simulink model "scara"  (R2015a)
settings: Solver=ode1  StartTime=0.0  StopTime=Inf  FixedStep=0.001  RelTol=1e-3
PostLoadFcn:
  | , if any(exist('dsrtsu_mdlpostloadfcn', 'file') == [2, 3, 6]), try dsrtsu_mdlpostloadfcn('Execute', bdroot); catch fprintf('Error in PostLoadFcn (dsrtsu_mdlpostloadfcn) for model "%s":\n %s\n', bdroot, lasterr); end, end,
libraries: rtilib1104 x9, simulink x6, simulink_extras x4
settings Model: DSRTSU_INTERNAL_RTI_VER=460  DSRTSU_INTERNAL_RTI_TYPE=rti1104  DSRTSU_INTERNAL_RTIFPGA=50  Creator=k21c900a  LastModifiedBy=k21c900a
settings OptimizationCC: BlockReduction=off  OptimizeBlockIOStorage=off  BufferReuse=off  GlobalBufferReuse=off  ExpressionFolding=off  LocalBlockOutputs=off
settings HardwareCC: ProdIntDivRoundTo=Zero  ProdEndianess=BigEndian  ProdHWDeviceType=Generic->Custom  TargetIntDivRoundTo=Zero  TargetEndianess=BigEndian  TargetHWDeviceType=Generic->Custom
settings RTWCC: SystemTargetFile=rti1104.tlc  MakeCommand=make_rti  TemplateMakefile=rti1104.tmf  Description=dSPACE DS1104 Hardware Platform
settings STFCustomTargetCC: GenerateSampleERTMain=off  ParMdlRefBuildCompliant=on  GeneratePreprocessorConditionals=Disable all  ERTCustomFileBanners=off  SupportNonInlinedSFcns=on  SupportVariableSizeSignals=off  MATLABClassNameForMDSCustomization=Simulink.SoftwareTarget.GRTCustomization  GRTInterface=on  SystemTargetFile=rti1104.tlc
settings GRTTargetCC: CompOptLevelCompliant=off  ConcurrentExecutionCompliant=off  CombineOutputUpdateFcns=off  MatFileLogging=off  CPPClassGenCompliant=off  GRTInterface=on  ExtModeMexFile=noextcomm

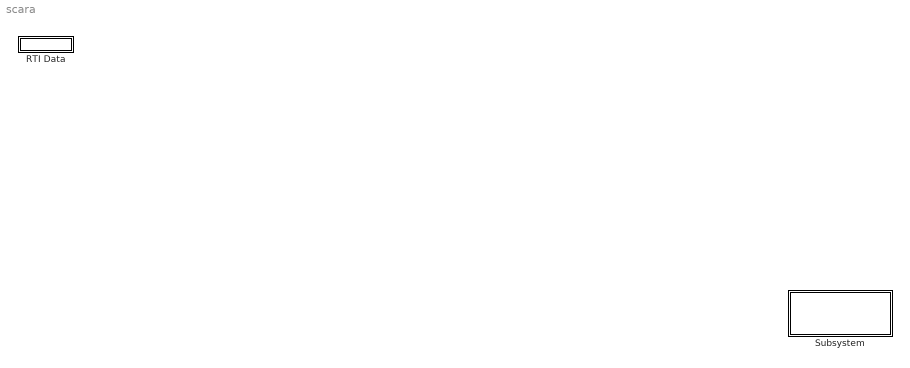
== system scara ==
  RTI Data : Subsystem  Tag=struct('RTIDataServer',struct('RTIDataServerVs','2','RTIModelDescription','struct(''main'',''scara'',''sub'','''',''isMp'',0)'))  LoadFcn="if exist('rtidc'), try,  rtidc('DataHostBlockClbLoad', gcbh); catch, disp(['Warning: ''LoadFcn'' for RTI Data block failed: ' lasterr]); end, end,"  mask(RTI_DATA_HOST){}
      mask help:
      | RTI Data Block.
      | This block is used by RTI to store internal model-dependent data.
      | Please keep this block on the root level of the model. Deleting this block will result in data loss.
      |
      | NEVER DELETE OR COPY THIS BLOCK!
      settings: CopyFcn="if exist('rtidc'), try,  rtidc('DataHostBlockClbCopy', gcbh); catch, disp(['Warning: ''CopyFcn'' for RTI Data block failed: ' lasterr]); end, end,"  DeleteFcn="if exist('rtidc'), try,  rtidc('DataHostBlockClbDelete', gcbh); catch, disp(['Warning: ''DeleteFcn'' for RTI Data block failed: ' lasterr]); end, end,"  ModelCloseFcn="if exist('rtidc'), try,  rtidc('DataHostBlockClbModelClose', gcbh); catch, disp(['Warning: ''ModelCloseFcn'' for RTI Data block failed: ' lasterr]); end, end,"  PreSaveFcn="if exist('rtidc'), try,  rtidc('DataHostBlockClbPreSave', gcbh); catch, disp(['Warning: ''PreSaveFcn'' for RTI Data block failed: ' lasterr]); end, end,"  PostSaveFcn="if exist('rtidc'), try,  rtidc('DataHostBlockClbPostSave', gcbh); catch, disp(['Warning: ''PostSaveFcn'' for RTI Data block failed: ' lasterr]); end, end,"  NameChangeFcn="if exist('rtidc'), try,  rtidc('DataHostBlockClbNameChange', gcbh); catch, disp(['Warning: ''NameChangeFcn'' for RTI Data block failed: ' lasterr]); end, end,"
      mask Help:
      | RTI Data Block.
      | This block is used by RTI to store internal model-dependent data.
      | Please keep this block on the root level of the model. Deleting this block will result in data loss.
      | 
      | NEVER DELETE OR COPY THIS BLOCK!
      mask Display:
      | text(0.5, 0.5, 'RTI Data', 'HorizontalAlignment', 'center');
      | plot([1 0]);
  Subsystem : Subsystem

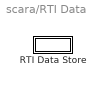
== system scara/RTI Data ==
  RTI Data Store : Subsystem  Tag="struct('private',struct('version',struct('dsVer',uint32(2),'dsVerCreation',uint32(2),'RTI',struct('ver','7.4','type','RTI1104')),'access',struct('type','Model','isPerm',1,'created',['18-Nov-2021 09:18:31'],'modified',['25-Nov-2021 10:31:28'],'location','')),'public',struct('main',struct('data',[]),'sub',struct('name',{{'scara'}},'data',{{struct('TH',struct('thTaskInfo',struct('taskType',{'TIMER','HWINT','TMRINT','SWINT','GLINT'},'tasksNumOf',{1,0,0,0,0},'srcIds',{{'TIMERA'},{},{},{},{}},'taskNames',{{['Timer Task 1']},{},{},{},{}})),'th_tc',struct('dataType','TASK','taskGroupId','','taskGroupList',{{}},'taskSchedulingPolicy','FCFS','taskType','TIMER','blkh',-1,'srcId','TIMERA','srcSgnName',['Timer A interrupt'],'srcCpuName','','taskName',['Timer Task 1  [0.001] s'],'taskNameDisplayExt','','smplTime',0.001,'smplTimeOffs',0,'hasFixedPriority',0,'priority',1,'hasFixedOvc',0,'ovcType',1,'ovcMax',1),'tc_th',struct('dataType','TASK','taskGroupId','','taskGroupList',{{}},'taskSchedulingPolicy','FCFS','taskType','TIMER','blkh',-1,'srcId','TIMERA','srcSgnName',['Timer A interrupt'],'srcCpuName','','taskName',['Timer Task 1  [0.001] s'],'taskNameDisplayExt','','smplTime',0.001,'smplTimeOffs',0,'hasFixedPriority',0,'priority',1,'hasFixedOvc',0,'ovcType',1,'ovcMax',1))}})))"  mask(RTI_DATA_STORE){}
      mask help:
      | RTI Data Store Block. This block is used by RTI to store internal model dependent data. Deleting this block will result in data loss.
      |
      | NEVER DELETE, COPY, OR MODIFY THIS BLOCK!
      mask Help:
      | RTI Data Store Block. This block is used by RTI to store internal model dependent data. Deleting this block will result in data loss.
      | 
      | NEVER DELETE, COPY, OR MODIFY THIS BLOCK!
      mask Display: text(0.5, 0.5, ' ', 'HorizontalAlignment', 'center');

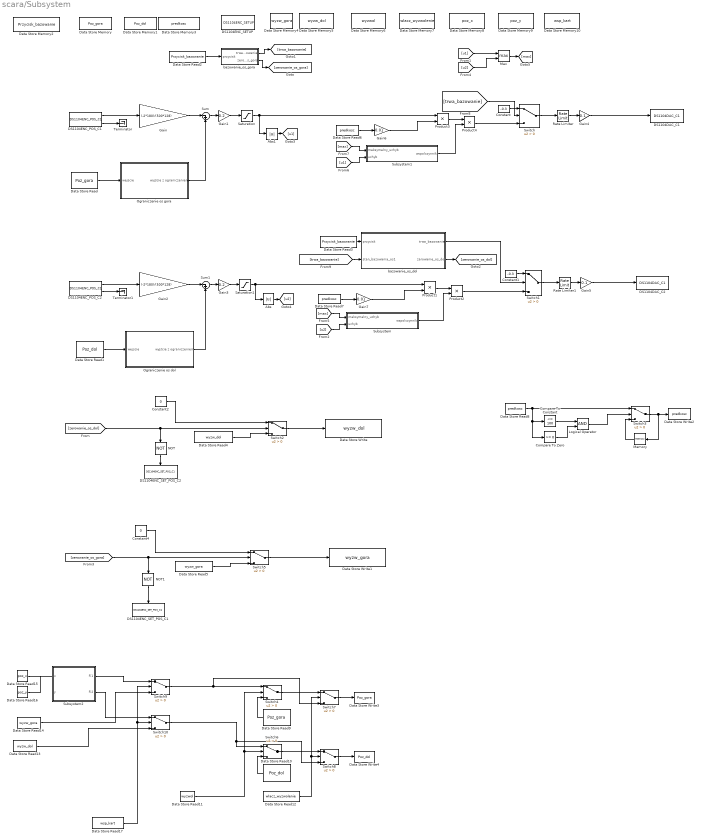
== system scara/Subsystem ==
  Abs : Abs
  Abs1 : Abs
  Compare To Constant : simulink/Logic and Bit Operations/Compare To Constant  relop=<=  const=100  OutDataTypeStr=boolean
  Compare To Zero : simulink/Logic and Bit Operations/Compare To Zero  relop=>=  OutDataTypeStr=boolean
  Constant : Constant  Value=-0.3
  Constant1 : Constant  Value=-0.3
  Constant2 : Constant  Value=0
  Constant4 : Constant  Value=0
  DS1104DAC_C1 : rtilib1104/DS1104 MASTER PPC/DS1104DAC_C1  ChannelNo=1  InitValue=0  TermMode=0  TermValue=0  Reserved1=[]  Reserved2=[]  Reserved3=[]  Reserved4=[]  DialogFcn=gui1104dac  UnitName={ 'DS1104DAC_C'}  UnitValues={ 1 }  DSProperties=struct('RTI',struct('Version',uint32(1),'BlockType',struct('isSLSource',uint8(0),'isSLSink',uint8(1),'isHWSource',uint8(0),'isHWSink',uint8(1),'isSetup',uint8(0),'isInline',uint8(1),'isNonInline',uint8(0),'isInterrupt',uint8(0),'isChannelwise',uint8(1)),'IOBoardType','DS1104MASTER','UnitType','DAC','Identifier','DAC','DialogType','ML','BlockSet','NONE','SlaveProcessor','NONE'))
  DS1104DAC_C2 : rtilib1104/DS1104 MASTER PPC/DS1104DAC_C1  ChannelNo=2  InitValue=0  TermMode=0  TermValue=0  Reserved1=[]  Reserved2=[]  Reserved3=[]  Reserved4=[]  DialogFcn=gui1104dac  UnitName={ 'DS1104DAC_C'}  UnitValues={2}  DSProperties=struct('RTI',struct('Version',uint32(1),'BlockType',struct('isSLSource',uint8(0),'isSLSink',uint8(1),'isHWSource',uint8(0),'isHWSink',uint8(1),'isSetup',uint8(0),'isInline',uint8(1),'isNonInline',uint8(0),'isInterrupt',uint8(0),'isChannelwise',uint8(1)),'IOBoardType','DS1104MASTER','UnitType','DAC','Identifier','DAC','DialogType','ML','BlockSet','NONE','SlaveProcessor','NONE'))
  DS1104ENC_POS_C1 : rtilib1104/DS1104 MASTER PPC/DS1104ENC_POS_C1  ChannelNo=1  PosValue=0  Reserved1=[]  Reserved2=[]  Reserved3=[]  Reserved4=[]  DialogFcn=gui1104enc_pos  UnitName={'DS1104ENC_POS_C'}  UnitValues={ 1 }  DSProperties=struct('RTI',struct('Version',uint32(1),'BlockType',struct('isSLSource',uint8(1),'isSLSink',uint8(0),'isHWSource',uint8(1),'isHWSink',uint8(0),'isSetup',uint8(0),'isInline',uint8(1),'isNonInline',uint8(0),'isInterrupt',uint8(0),'isChannelwise',uint8(1)),'IOBoardType','DS1104MASTER','UnitType','ENC','Identifier','ENCPOSCH','DialogType','ML','BlockSet','NONE','SlaveProcessor','NONE'))
  DS1104ENC_POS_C2 : rtilib1104/DS1104 MASTER PPC/DS1104ENC_POS_C1  ChannelNo=2  PosValue=0  Reserved1=[]  Reserved2=[]  Reserved3=[]  Reserved4=[]  DialogFcn=gui1104enc_pos  UnitName={'DS1104ENC_POS_C'}  UnitValues={2}  DSProperties=struct('RTI',struct('Version',uint32(1),'BlockType',struct('isSLSource',uint8(1),'isSLSink',uint8(0),'isHWSource',uint8(1),'isHWSink',uint8(0),'isSetup',uint8(0),'isInline',uint8(1),'isNonInline',uint8(0),'isInterrupt',uint8(0),'isChannelwise',uint8(1)),'IOBoardType','DS1104MASTER','UnitType','ENC','Identifier','ENCPOSCH','DialogType','ML','BlockSet','NONE','SlaveProcessor','NONE'))
  DS1104ENC_SETUP : rtilib1104/DS1104 MASTER PPC/DS1104ENC_SETUP  Reserved1=[]  Reserved2=[]  Reserved3=[]  Reserved4=[]  DialogFcn=gui1104enc_setup  UnitName={'DS1104ENC_SETUP'}  UnitValues={ [] }  DSProperties=struct('RTI',struct('Version',uint32(1),'BlockType',struct('isSLSource',uint8(0),'isSLSink',uint8(0),'isHWSource',uint8(0),'isHWSink',uint8(0),'isSetup',uint8(0),'isInline',uint8(1),'isNonInline',uint8(0),'isInterrupt',uint8(0),'isChannelwise',uint8(0)),'IOBoardType','DS1104MASTER','UnitType','ENC','Identifier','ENCSETUP','DialogType','ML','BlockSet','NONE','SlaveProcessor','NONE'))
      settings: SignalType=[0 0]
  DS1104ENC_SET_POS_C1 : rtilib1104/DS1104 MASTER PPC/DS1104ENC_SET_POS_C1  ChannelNo=1  PosValue=0  Reserved1=[]  Reserved2=[]  Reserved3=[]  Reserved4=[]  DialogFcn=gui1104enc_set_pos  UnitName={'DS1104ENC_SET_POS_C'}  UnitValues={ 1 }  DSProperties=struct('RTI',struct('Version',uint32(1),'BlockType',struct('isSLSource',uint8(0),'isSLSink',uint8(1),'isHWSource',uint8(0),'isHWSink',uint8(1),'isSetup',uint8(0),'isInline',uint8(1),'isNonInline',uint8(0),'isInterrupt',uint8(0),'isChannelwise',uint8(1)),'IOBoardType','DS1104MASTER','UnitType','ENC','Identifier','ENCRESET','DialogType','ML','BlockSet','NONE','SlaveProcessor','NONE'))
  DS1104ENC_SET_POS_C2 : rtilib1104/DS1104 MASTER PPC/DS1104ENC_SET_POS_C1  ChannelNo=2  PosValue=0  Reserved1=[]  Reserved2=[]  Reserved3=[]  Reserved4=[]  DialogFcn=gui1104enc_set_pos  UnitName={'DS1104ENC_SET_POS_C'}  UnitValues={ 2 }  DSProperties=struct('RTI',struct('Version',uint32(1),'BlockType',struct('isSLSource',uint8(0),'isSLSink',uint8(1),'isHWSource',uint8(0),'isHWSink',uint8(1),'isSetup',uint8(0),'isInline',uint8(1),'isNonInline',uint8(0),'isInterrupt',uint8(0),'isChannelwise',uint8(1)),'IOBoardType','DS1104MASTER','UnitType','ENC','Identifier','ENCRESET','DialogType','ML','BlockSet','NONE','SlaveProcessor','NONE'))
  Data Store Memory : DataStoreMemory  DataStoreName=Poz_gora  ReadBeforeWriteMsg=warning  WriteAfterWriteMsg=warning  WriteAfterReadMsg=warning
  Data Store Memory1 : DataStoreMemory  DataStoreName=Poz_dol  ReadBeforeWriteMsg=warning  WriteAfterWriteMsg=warning  WriteAfterReadMsg=warning
  Data Store Memory10 : DataStoreMemory  DataStoreName=wsp_kart  ReadBeforeWriteMsg=warning  WriteAfterWriteMsg=warning  WriteAfterReadMsg=warning
  Data Store Memory2 : DataStoreMemory  DataStoreName=Przycisk_bazowanie  ReadBeforeWriteMsg=warning  WriteAfterWriteMsg=warning  WriteAfterReadMsg=warning
  Data Store Memory3 : DataStoreMemory  DataStoreName=predkosc  ReadBeforeWriteMsg=warning  WriteAfterWriteMsg=warning  WriteAfterReadMsg=warning
  Data Store Memory4 : DataStoreMemory  DataStoreName=wyzw_gora  ReadBeforeWriteMsg=warning  WriteAfterWriteMsg=warning  WriteAfterReadMsg=warning
  Data Store Memory5 : DataStoreMemory  DataStoreName=wyzw_dol  ReadBeforeWriteMsg=warning  WriteAfterWriteMsg=warning  WriteAfterReadMsg=warning
  Data Store Memory6 : DataStoreMemory  DataStoreName=wyzwol  ReadBeforeWriteMsg=warning  WriteAfterWriteMsg=warning  WriteAfterReadMsg=warning
  Data Store Memory7 : DataStoreMemory  DataStoreName=wlacz_wyzwolenie  ReadBeforeWriteMsg=warning  WriteAfterWriteMsg=warning  WriteAfterReadMsg=warning
  Data Store Memory8 : DataStoreMemory  DataStoreName=poz_x  ReadBeforeWriteMsg=warning  WriteAfterWriteMsg=warning  WriteAfterReadMsg=warning
  Data Store Memory9 : DataStoreMemory  DataStoreName=poz_y  ReadBeforeWriteMsg=warning  WriteAfterWriteMsg=warning  WriteAfterReadMsg=warning
  Data Store Read : DataStoreRead  DataStoreName=Poz_gora
  Data Store Read1 : DataStoreRead  DataStoreName=Poz_dol
  Data Store Read10 : DataStoreRead  DataStoreName=Poz_dol
  Data Store Read11 : DataStoreRead  DataStoreName=wyzwol
  Data Store Read12 : DataStoreRead  DataStoreName=wlacz_wyzwolenie
  Data Store Read13 : DataStoreRead  DataStoreName=wyzw_dol
  Data Store Read14 : DataStoreRead  DataStoreName=wyzw_gora
  Data Store Read15 : DataStoreRead  DataStoreName=poz_x
  Data Store Read16 : DataStoreRead  DataStoreName=poz_y
  Data Store Read17 : DataStoreRead  DataStoreName=wsp_kart
  Data Store Read2 : DataStoreRead  DataStoreName=Przycisk_bazowanie
  Data Store Read3 : DataStoreRead  DataStoreName=Przycisk_bazowanie
  Data Store Read4 : DataStoreRead  DataStoreName=wyzw_dol
  Data Store Read5 : DataStoreRead  DataStoreName=wyzw_gora
  Data Store Read6 : DataStoreRead  DataStoreName=predkosc
  Data Store Read7 : DataStoreRead  DataStoreName=predkosc
  Data Store Read8 : DataStoreRead  DataStoreName=predkosc
  Data Store Read9 : DataStoreRead  DataStoreName=Poz_gora
  Data Store Write : DataStoreWrite  DataStoreName=wyzw_dol
  Data Store Write1 : DataStoreWrite  DataStoreName=wyzw_gora
  Data Store Write2 : DataStoreWrite  DataStoreName=predkosc
  Data Store Write3 : DataStoreWrite  DataStoreName=Poz_gora
  Data Store Write4 : DataStoreWrite  DataStoreName=Poz_dol
  Gain : Gain  Gain=(-2*180)/(500*128)
  Gain1 : Gain  Gain=0.2
  Gain2 : Gain  Gain=(-2*180)/(500*128)
  Gain3 : Gain  Gain=0.2
  Gain4 : Gain  Gain=0.1
  Gain5 : Gain  Gain=0.1
  Gain6 : Gain  Gain=0.01
  Gain7 : Gain  Gain=0.01
  Logical Operator : Logic  AllPortsSameDT=off  OutDataTypeStr=boolean
  Max : MinMax  Function=max  Inputs=2
  Memory : Memory
  NOT : Logic  Operator=NOT  IconShape=distinctive  AllPortsSameDT=off  OutDataTypeStr=boolean
  NOT1 : Logic  Operator=NOT  IconShape=distinctive  AllPortsSameDT=off  OutDataTypeStr=boolean
  Ograniczenie os dol : Subsystem
  Ograniczenie os gora : Subsystem
  Product{1..4} (4 alike) : Product
  Rate Limiter : RateLimiter  RisingSlewLimit=50  FallingSlewLimit=-50  SampleTimeMode=inherited
  Rate Limiter1 : RateLimiter  RisingSlewLimit=50  FallingSlewLimit=-50  SampleTimeMode=inherited
  Saturation : Saturate  UpperLimit=3  LowerLimit=-3
  Saturation1 : Saturate  UpperLimit=3  LowerLimit=-3
  Subsystem : Subsystem
  Subsystem1 : Subsystem
  Subsystem2 : Subsystem
  Sum : Sum  Inputs=|-+
  Sum1 : Sum  Inputs=|-+
  Switch{,1..10} (11 alike) : Switch  Criteria=u2 > Threshold
  Terminator : Terminator
  Terminator1 : Terminator
  bazowanie_os_dol : Subsystem
  bazowanie_os_gora : Subsystem
  wires:
  Data Store Read2/1 -> bazowanie_os_gora/1(przycisk)
  Data Store Read4/1 -> Switch2/3
  Switch2/1 -> Data Store Write/1
  [zerowanie_os_dol] -> Switch2/2, NOT/1
  Constant2/1 -> Switch2/1
  NOT/1 -> DS1104ENC_SET_POS_C2/Trigger
  bazowanie_os_gora/2(zerowanie_os_gora) -> [zerowanie_os_gora]
  bazowanie_os_gora/1(trwa_bazowanie) -> [trwa_bazowanie]
  Switch5/1 -> Data Store Write1/1
  Constant4/1 -> Switch5/1
  Data Store Read5/1 -> Switch5/3
  [zerowanie_os_gora] -> NOT1/1, Switch5/2
  NOT1/1 -> DS1104ENC_SET_POS_C1/Trigger
  DS1104ENC_POS_C1/2 -> Terminator/1
  DS1104ENC_POS_C1/1 -> Gain/1
  Gain/1 -> Sum/1
  Sum/1 -> Gain1/1
  Rate Limiter/1 -> Gain4/1
  DS1104ENC_POS_C2/2 -> Terminator1/1
  DS1104ENC_POS_C2/1 -> Gain2/1
  Gain2/1 -> Sum1/1
  Sum1/1 -> Gain3/1
  Gain3/1 -> Saturation1/1
  Rate Limiter1/1 -> Gain5/1
  Data Store Read/1 -> Ograniczenie os gora/1(wejscie)
  Ograniczenie os gora/1(wyjście z ograniczeniem) -> Sum/2
  Data Store Read1/1 -> Ograniczenie os dol/1(wejscie)
  Ograniczenie os dol/1(wyjście z ograniczeniem) -> Sum1/2
  Gain4/1 -> DS1104DAC_C1/1
  Gain5/1 -> DS1104DAC_C2/1
  Gain1/1 -> Saturation/1
  Constant/1 -> Switch/1
  Switch/1 -> Rate Limiter/1
  Constant1/1 -> Switch1/1
  bazowanie_os_dol/1(trwa_bazowanie) -> Switch1/2
  Switch1/1 -> Rate Limiter1/1
  Data Store Read3/1 -> bazowanie_os_dol/1(przycisk)
  bazowanie_os_dol/2(zarowanie_os_dol) -> [zerowanie_os_dol]
  Abs1/1 -> [u1]
  Abs/1 -> [u2]
  Product1/1 -> Product2/1
  Saturation1/1 -> Product1/1, Abs/1
  Subsystem/1(wspolczynnik) -> Product2/2
  [u2] -> Subsystem/2(uchyb)
  Product2/1 -> Switch1/3
  Data Store Read7/1 -> Gain7/1
  Gain7/1 -> Product1/2
  [max] -> Subsystem/1(maksymalny_uchyb)
  Product3/1 -> Product4/1
  Saturation/1 -> Product3/1, Abs1/1
  Subsystem1/1(wspolczynnik) -> Product4/2
  [u1] -> Subsystem1/2(uchyb)
  Product4/1 -> Switch/3
  Data Store Read6/1 -> Gain6/1
  Gain6/1 -> Product3/2
  [max] -> Subsystem1/1(maksymalny_uchyb)
  [trwa_bazowanie] -> Switch/2
  [trwa_bazowanie] -> bazowanie_os_dol/2(stan_bazowania_os1)
  [u1] -> Max/1
  [u2] -> Max/2
  Max/1 -> [max]
  Switch3/1 -> Memory/1, Data Store Write2/1
  Memory/1 -> Switch3/3
  Data Store Read8/1 -> Compare To Constant/1, Compare To Zero/1, Switch3/1
  Compare To Constant/1 -> Logical Operator/1
  Compare To Zero/1 -> Logical Operator/2
  Logical Operator/1 -> Switch3/2
  Data Store Read11/1 -> Switch6/2, Switch4/2
  Switch4/1 -> Switch7/1
  Switch6/1 -> Switch8/1
  Data Store Read12/1 -> Switch8/2, Switch7/2
  Data Store Read9/1 -> Switch4/3
  Data Store Read10/1 -> Switch6/3
  Switch7/1 -> Data Store Write3/1
  Switch8/1 -> Data Store Write4/1
  Switch9/1 -> Switch7/3, Switch4/1
  Switch10/1 -> Switch6/1, Switch8/3
  Data Store Read15/1 -> ?
  Data Store Read16/1 -> ?
  Data Store Read17/1 -> Switch9/2, Switch10/2
  Data Store Read14/1 -> Switch9/3
  Data Store Read13/1 -> Switch10/3
  Subsystem2/1(Fi1) -> Switch9/1
  Subsystem2/2(Fi2) -> Switch10/1

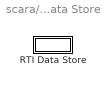
== system scara/RTI Data/RTI Data Store ==
  RTI Data Store : Subsystem  mask(RTI_DATA_STORE){}
      mask help:
      | RTI Data Store Block. This block is used by RTI to store internal model dependent data. Deleting this block will result in data loss.
      |
      | NEVER DELETE, COPY, OR MODIFY THIS BLOCK!
      mask Help:
      | RTI Data Store Block. This block is used by RTI to store internal model dependent data. Deleting this block will result in data loss.
      | 
      | NEVER DELETE, COPY, OR MODIFY THIS BLOCK!
      mask Display: text(0.5, 0.5, ' ', 'HorizontalAlignment', 'center');

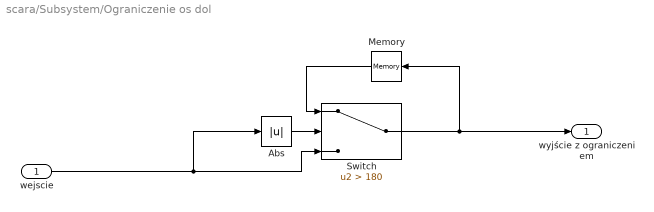
== system scara/Subsystem/Ograniczenie os dol ==
  wejscie : Inport
  Abs : Abs
  Memory : Memory
  Switch : Switch  Criteria=u2 > Threshold  Threshold=180
  wyjście z ograniczeniem : Outport
  wires:
  Memory/1 -> Switch/1
  Switch/1 -> Memory/1, wyjście z ograniczeniem/1
  Abs/1 -> Switch/2
  wejscie/1 -> Abs/1, Switch/3

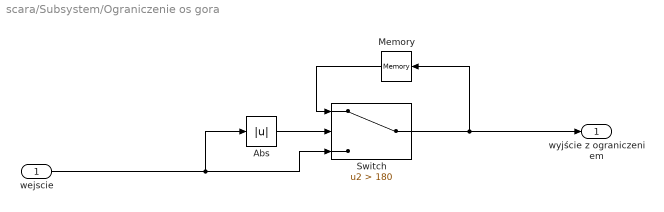
== system scara/Subsystem/Ograniczenie os gora ==
  wejscie : Inport
  Abs : Abs
  Memory : Memory
  Switch : Switch  Criteria=u2 > Threshold  Threshold=180
  wyjście z ograniczeniem : Outport
  wires:
  Memory/1 -> Switch/1
  Switch/1 -> Memory/1, wyjście z ograniczeniem/1
  Abs/1 -> Switch/2
  wejscie/1 -> Abs/1, Switch/3

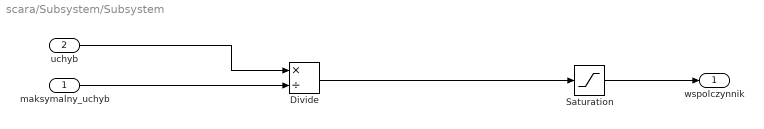
== system scara/Subsystem/Subsystem ==
  maksymalny_uchyb : Inport
  uchyb : Inport  Port=2
  Divide : Product  Inputs=*/
  Saturation : Saturate  UpperLimit=1  LowerLimit=0.01
  wspolczynnik : Outport
  wires:
  Saturation/1 -> wspolczynnik/1
  uchyb/1 -> Divide/1
  maksymalny_uchyb/1 -> Divide/2
  Divide/1 -> Saturation/1

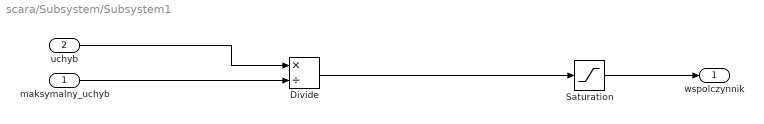
== system scara/Subsystem/Subsystem1 ==
  maksymalny_uchyb : Inport
  uchyb : Inport  Port=2
  Divide : Product  Inputs=*/
  Saturation : Saturate  UpperLimit=1  LowerLimit=0.01
  wspolczynnik : Outport
  wires:
  Saturation/1 -> wspolczynnik/1
  uchyb/1 -> Divide/1
  maksymalny_uchyb/1 -> Divide/2
  Divide/1 -> Saturation/1

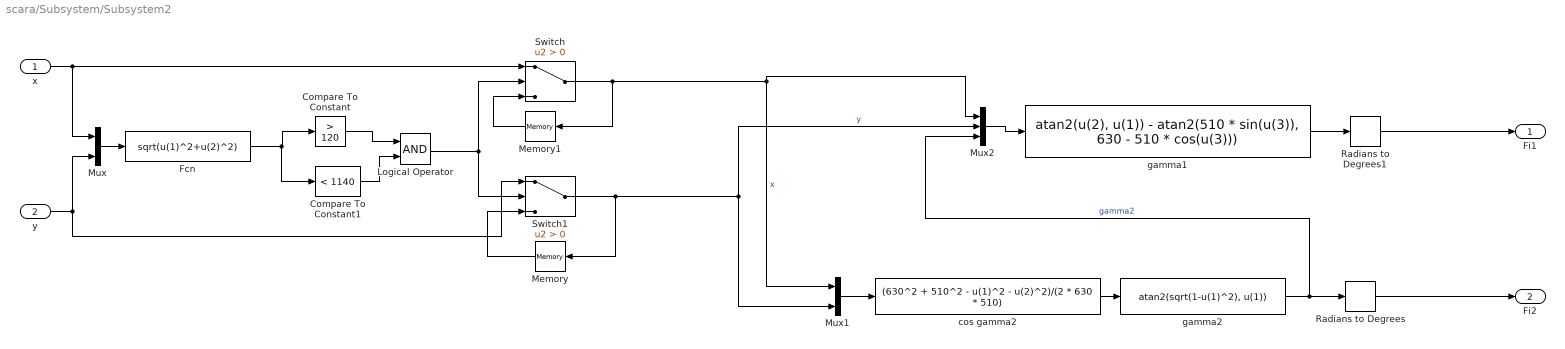
== system scara/Subsystem/Subsystem2 ==
  x : Inport
  y : Inport  Port=2
  Compare To Constant : simulink/Logic and Bit Operations/Compare To Constant  relop=>  const=120  OutDataTypeStr=boolean
  Compare To Constant1 : simulink/Logic and Bit Operations/Compare To Constant  relop=<  const=1140  OutDataTypeStr=boolean
  Fcn : Fcn  Expr=sqrt(u(1)^2+u(2)^2)
  Logical Operator : Logic  AllPortsSameDT=off  OutDataTypeStr=boolean
  Memory : Memory
  Memory1 : Memory
  Mux : Mux  Inputs=2
  Mux1 : Mux  Inputs=2
  Mux2 : Mux  Inputs=3
  Radians to Degrees : simulink_extras/Transformations/Radians to Degrees
  Radians to Degrees1 : simulink_extras/Transformations/Radians to Degrees
  Switch : Switch  Criteria=u2 > Threshold
  Switch1 : Switch  Criteria=u2 > Threshold
  "cos gamma2 " : Fcn  Expr=(630^2 + 510^2 - u(1)^2 - u(2)^2)/(2 * 630 * 510)
  gamma1 : Fcn  Expr=atan2(u(2), u(1)) - atan2(510 * sin(u(3)), 630 - 510 * cos(u(3)))
  "gamma2 " : Fcn  Expr=atan2(sqrt(1-u(1)^2), u(1))
  Fi1 : Outport
  Fi2 : Outport  Port=2
  wires:
  "gamma2 "/1 -> Radians to Degrees/1, Mux2/3  "gamma2"
  Mux2/1 -> gamma1/1
  Radians to Degrees1/1 -> Fi1/1
  Switch/1 -> Memory1/1, Mux2/1, Mux1/1  "x"
  "cos gamma2 "/1 -> "gamma2 "/1
  Radians to Degrees/1 -> Fi2/1
  Mux1/1 -> "cos gamma2 "/1
  Switch1/1 -> Memory/1, Mux1/2, Mux2/2  "y"
  gamma1/1 -> Radians to Degrees1/1
  Mux/1 -> Fcn/1
  y/1 -> Switch1/1, Mux/2
  x/1 -> Switch/1, Mux/1
  Fcn/1 -> Compare To Constant1/1, Compare To Constant/1
  Compare To Constant/1 -> Logical Operator/1
  Compare To Constant1/1 -> Logical Operator/2
  Logical Operator/1 -> Switch1/2, Switch/2
  Memory/1 -> Switch1/3
  Memory1/1 -> Switch/3

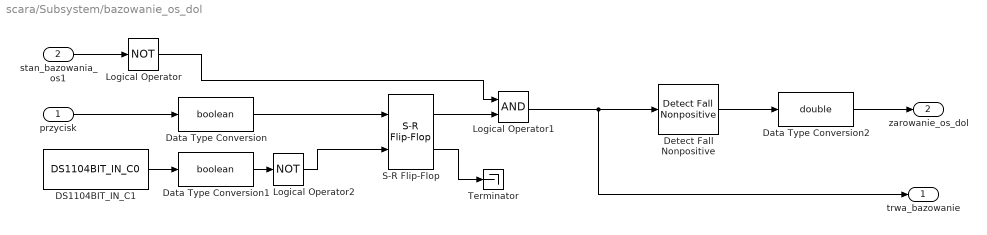
== system scara/Subsystem/bazowanie_os_dol ==
  przycisk : Inport
  stan_bazowania_os1 : Inport  Port=2
  DS1104BIT_IN_C1 : rtilib1104/DS1104 MASTER PPC/DS1104BIT_IN_C0  ChannelNo=1  Reserved1=[]  Reserved2=[]  Reserved3=[]  Reserved4=[]  DialogFcn=gui1104bit_in  UnitName={'DS1104BIT_IN_C'}  UnitValues={ 1 }  DSProperties=struct('RTI',struct('Version',uint32(1),'BlockType',struct('isSLSource',uint8(1),'isSLSink',uint8(0),'isHWSource',uint8(1),'isHWSink',uint8(0),'isSetup',uint8(0),'isInline',uint8(1),'isNonInline',uint8(0),'isInterrupt',uint8(0),'isChannelwise',uint8(1)),'IOBoardType','DS1104MASTER','UnitType','BIT','Identifier','BITINCH','DialogType','ML','BlockSet','NONE','SlaveProcessor','NONE'))
  Data Type Conversion : DataTypeConversion  OutDataTypeStr=boolean
  Data Type Conversion1 : DataTypeConversion  OutDataTypeStr=boolean
  Data Type Conversion2 : DataTypeConversion  OutDataTypeStr=double
  Detect Fall Nonpositive : simulink/Logic and Bit Operations/Detect Fall Nonpositive  vinit=0  OutDataTypeStr=boolean
  Logical Operator : Logic  Operator=NOT  AllPortsSameDT=off  OutDataTypeStr=boolean
  Logical Operator1 : Logic  AllPortsSameDT=off  OutDataTypeStr=boolean
  Logical Operator2 : Logic  Operator=NOT  AllPortsSameDT=off  OutDataTypeStr=boolean
  S-R Flip-Flop : simulink_extras/Flip Flops/S-R Flip-Flop  initial_condition=0
  Terminator : Terminator
  trwa_bazowanie : Outport
  zarowanie_os_dol : Outport  Port=2
  wires:
  S-R Flip-Flop/2 -> Terminator/1
  Detect Fall Nonpositive/1 -> Data Type Conversion2/1
  stan_bazowania_os1/1 -> Logical Operator/1
  Logical Operator/1 -> Logical Operator1/1
  DS1104BIT_IN_C1/1 -> Data Type Conversion1/1
  Logical Operator2/1 -> S-R Flip-Flop/2
  S-R Flip-Flop/1 -> Logical Operator1/2
  przycisk/1 -> Data Type Conversion/1
  Logical Operator1/1 -> Detect Fall Nonpositive/1, trwa_bazowanie/1
  Data Type Conversion/1 -> S-R Flip-Flop/1
  Data Type Conversion1/1 -> Logical Operator2/1
  Data Type Conversion2/1 -> zarowanie_os_dol/1

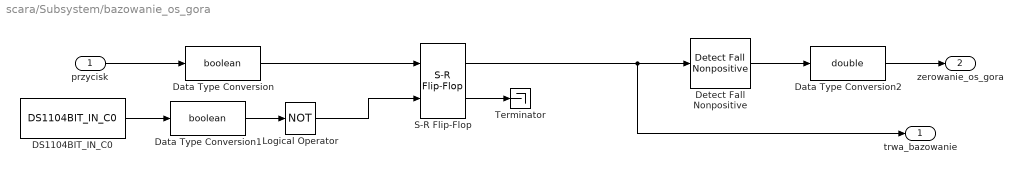
== system scara/Subsystem/bazowanie_os_gora ==
  przycisk : Inport
  DS1104BIT_IN_C0 : rtilib1104/DS1104 MASTER PPC/DS1104BIT_IN_C0  ChannelNo=0  Reserved1=[]  Reserved2=[]  Reserved3=[]  Reserved4=[]  DialogFcn=gui1104bit_in  UnitName={'DS1104BIT_IN_C'}  UnitValues={ 0 }  DSProperties=struct('RTI',struct('Version',uint32(1),'BlockType',struct('isSLSource',uint8(1),'isSLSink',uint8(0),'isHWSource',uint8(1),'isHWSink',uint8(0),'isSetup',uint8(0),'isInline',uint8(1),'isNonInline',uint8(0),'isInterrupt',uint8(0),'isChannelwise',uint8(1)),'IOBoardType','DS1104MASTER','UnitType','BIT','Identifier','BITINCH','DialogType','ML','BlockSet','NONE','SlaveProcessor','NONE'))
  Data Type Conversion : DataTypeConversion  OutDataTypeStr=boolean
  Data Type Conversion1 : DataTypeConversion  OutDataTypeStr=boolean
  Data Type Conversion2 : DataTypeConversion  OutDataTypeStr=double
  Detect Fall Nonpositive : simulink/Logic and Bit Operations/Detect Fall Nonpositive  vinit=0  InputProcessing=Inherited  OutDataTypeStr=boolean
  Logical Operator : Logic  Operator=NOT  AllPortsSameDT=off  OutDataTypeStr=boolean
  S-R Flip-Flop : simulink_extras/Flip Flops/S-R Flip-Flop  initial_condition=0
  Terminator : Terminator
  trwa_bazowanie : Outport
  zerowanie_os_gora : Outport  Port=2
  wires:
  przycisk/1 -> Data Type Conversion/1
  S-R Flip-Flop/1 -> Detect Fall Nonpositive/1, trwa_bazowanie/1
  S-R Flip-Flop/2 -> Terminator/1
  Detect Fall Nonpositive/1 -> Data Type Conversion2/1
  DS1104BIT_IN_C0/1 -> Data Type Conversion1/1
  Logical Operator/1 -> S-R Flip-Flop/2
  Data Type Conversion/1 -> S-R Flip-Flop/1
  Data Type Conversion1/1 -> Logical Operator/1
  Data Type Conversion2/1 -> zerowanie_os_gora/1

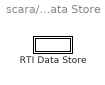
== system scara/RTI Data/RTI Data Store/RTI Data Store ==
  RTI Data Store : Subsystem  mask(RTI_DATA_STORE){}
      mask help:
      | RTI Data Store Block. This block is used by RTI to store internal model dependent data. Deleting this block will result in data loss.
      |
      | NEVER DELETE, COPY, OR MODIFY THIS BLOCK!
      mask Help:
      | RTI Data Store Block. This block is used by RTI to store internal model dependent data. Deleting this block will result in data loss.
      | 
      | NEVER DELETE, COPY, OR MODIFY THIS BLOCK!
      mask Display: text(0.5, 0.5, ' ', 'HorizontalAlignment', 'center');

== system scara/RTI Data/RTI Data Store/RTI Data Store/RTI Data Store ==
  RTI Data Store : Subsystem  mask(RTI_DATA_STORE){}
      mask help:
      | RTI Data Store Block. This block is used by RTI to store internal model dependent data. Deleting this block will result in data loss.
      |
      | NEVER DELETE, COPY, OR MODIFY THIS BLOCK!
      mask Help:
      | RTI Data Store Block. This block is used by RTI to store internal model dependent data. Deleting this block will result in data loss.
      | 
      | NEVER DELETE, COPY, OR MODIFY THIS BLOCK!
      mask Display: text(0.5, 0.5, ' ', 'HorizontalAlignment', 'center');

== system scara/RTI Data/RTI Data Store/RTI Data Store/RTI Data Store/RTI Data Store ==
